simulink model "s_mbd_02_06"  (R2020b)
settings: Solver=ode4  StartTime=0.0  StopTime=Endtime  FixedStep=1e-3  RelTol=1e-3
values from neighbouring files (symbols this model uses):
  D = 0.5    [m_mbd_02_04.m]    (also in m_mbd_02_06.m = 10)
  f = 20    [m_mbd_02_06.m]
  g = 9.81    [m_mbd_02_06.m]
  k = 100    [m_mbd_02_06.m]
  M = 10    [m_mbd_02_06.m]    (also in s_heatbalance.m = 1)
  p_cycle = 20    [m_mbd_02_06.m]
  p_width = 50    [m_mbd_02_06.m]
settings Model: Creator=005274  LastModifiedBy=005274

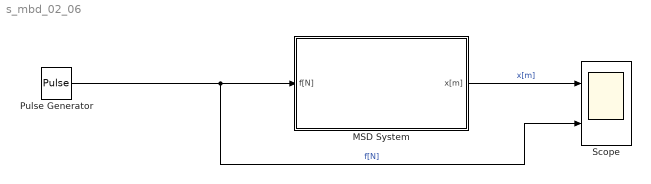
== system s_mbd_02_06 ==
  MSD System : Subsystem
  Pulse Generator : DiscretePulseGenerator  PulseType=Time based  Amplitude=f  Period=p_cycle  PulseWidth=p_width  PhaseDelay=10
  Scope : Scope  NumInputPorts=2
  wires:
  MSD System/1(x[m]) -> Scope/1  "x[m]"
  Pulse Generator/1 -> Scope/2, MSD System/1(f[N])  "f[N]"

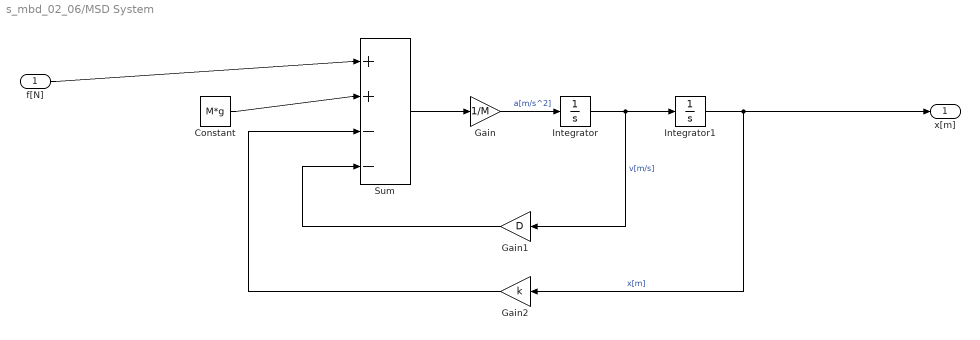
== system s_mbd_02_06/MSD System ==
  f[N] : Inport
  Constant : Constant  Value=M*g
  Gain : Gain  Gain=1/M
  Gain1 : Gain  Gain=D
  Gain2 : Gain  Gain=k
  Integrator : Integrator
  Integrator1 : Integrator  InitialCondition=M*g/k
  Sum : Sum  Inputs=|++--
  x[m] : Outport
  wires:
  f[N]/1 -> Sum/1
  Integrator/1 -> Gain1/1, Integrator1/1  "v[m/s]"
  Sum/1 -> Gain/1
  Gain/1 -> Integrator/1  "a[m/s^2]"
  Constant/1 -> Sum/2
  Gain1/1 -> Sum/4
  Integrator1/1 -> x[m]/1, Gain2/1  "x[m]"
  Gain2/1 -> Sum/3
